simulink model "FirstAttempt_ColdEarth"  (R2018b)
settings: Solver=VariableStepAuto  StartTime=0.0  StopTime=time  RelTol=1e-3
values from neighbouring files (symbols this model uses):
  A_side = 2 * A_front    (= 0.02)    [MultipleNodes.m]    (also in OneNode.m)
  eps_f = 1    [OneNode.m]
  eps_l = 0.81    [OneNode.m]
  Qa_e = 0    [OneNode.m]
  Qi = 0.2*Qdiss    (= 0.6)    [OneNode.m]
  Qir_e = Wir_e *A_front *eps_b*REF    (= 1.8144)    [OneNode.m]
  QS_e = 0    [OneNode.m]
  sigma = 5.67e-8    (= 5.67e-08)    [MultipleNodes.m]    (also in OneNode.m)
  Tds = 4    [MultipleNodes.m]    (also in OneNode.m)
  Tsc_c = T_sc(1,1)    [OneNode.m]
libraries: fl_lib x19, nesl_utility x8
settings Model: Creator=aloisia  LastModifiedBy=aloisia

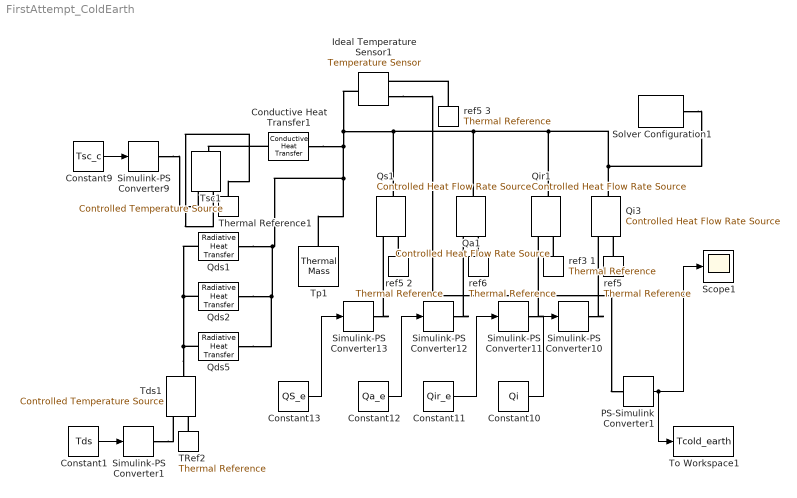
== system FirstAttempt_ColdEarth ==
  Conductive Heat Transfer1 : fl_lib/Thermal/Thermal Elements/Conductive Heat Transfer  area=0.005 m^2  thickness=0.01 m  th_cond=Gsc W/(m*K)  T_specify=off  T_priority=None  T=0 K  T_nominal_specify=off  T_nominal_unit=K  T_nominal_value=1  Q_specify=off  Q_priority=None  Q=0 J/s  Q_nominal_specify=off  Q_nominal_unit=W  Q_nominal_value=1
      settings: SourceProductName=Simscape
  Constant1 : Constant  Value=Tds
  Constant10 : Constant  Value=Qi
  Constant11 : Constant  Value=Qir_e
  Constant12 : Constant  Value=Qa_e
  Constant13 : Constant  Value=QS_e
  Constant9 : Constant  Value=Tsc_c
  Ideal Temperature Sensor1 : fl_lib/Thermal/Thermal Sensors/Temperature Sensor
  PS-Simulink Converter1 : nesl_utility/PS-Simulink Converter  PhysicalDomain=network_engine_domain  SubClassName=ps_output  LeftPortType=input  RightPortType=output  PseudoPeriodic=off  Frequencies=[]  Unit=1  AffineConversion=off
  Qa1 : fl_lib/Thermal/Thermal Sources/Controlled Heat Flow Rate Source
      settings: SourceProductName=Simscape
  Qds1 : fl_lib/Thermal/Thermal Elements/Radiative Heat Transfer  area=2*A_side m^2  rad_tr_coeff=sigma*eps_l W/(m^2*K^4)  T_specify=off  T_priority=None  T=0 K  T_nominal_specify=off  T_nominal_unit=K  T_nominal_value=1  Q_specify=off  Q_priority=None  Q=0 J/s  Q_nominal_specify=off  Q_nominal_unit=W  Q_nominal_value=1
      settings: SourceProductName=Simscape  SourceProductBaseCode=SS
  Qds2 : fl_lib/Thermal/Thermal Elements/Radiative Heat Transfer  area=A_front m^2  rad_tr_coeff=sigma*eps_f W/(m^2*K^4)  T_specify=off  T_priority=None  T=0 K  T_nominal_specify=off  T_nominal_unit=K  T_nominal_value=1  Q_specify=off  Q_priority=None  Q=0 J/s  Q_nominal_specify=off  Q_nominal_unit=W  Q_nominal_value=1
      settings: SourceProductName=Simscape  SourceProductBaseCode=SS
  Qds5 : fl_lib/Thermal/Thermal Elements/Radiative Heat Transfer  area=A_front m^2  rad_tr_coeff=sigma*eps_f W/(m^2*K^4)  T_specify=off  T_priority=None  T=0 K  T_nominal_specify=off  T_nominal_unit=K  T_nominal_value=1  Q_specify=off  Q_priority=None  Q=0 J/s  Q_nominal_specify=off  Q_nominal_unit=W  Q_nominal_value=1
      settings: SourceProductName=Simscape  SourceProductBaseCode=SS
  Qi3 : fl_lib/Thermal/Thermal Sources/Controlled Heat Flow Rate Source
      settings: SourceProductName=Simscape
  Qir1 : fl_lib/Thermal/Thermal Sources/Controlled Heat Flow Rate Source
      settings: SourceProductName=Simscape
  Qs1 : fl_lib/Thermal/Thermal Sources/Controlled Heat Flow Rate Source
      settings: SourceProductName=Simscape
  Scope1 : Scope
  Simulink-PS Converter{1,9..13} (6 alike) : nesl_utility/Simulink-PS Converter  PhysicalDomain=network_engine_domain  SubClassName=ps_input  LeftPortType=input  RightPortType=output  PseudoPeriodic=off  Frequencies=[]  NoiseDistribution=none  NoiseParameters=[]  Unit=1  AffineConversion=off  FilteringAndDerivatives=zero  SimscapeFilterOrder=1  InputFilterTimeConstant=0.001  UdotUserProvided=1
  Solver Configuration1 : nesl_utility/Solver Configuration  PhysicalDomain=network_engine_domain  SubClassName=solver  LeftPortType=input  RightPortType=generic  Tones=[]  Harmonics=[]  SimulateNoise=off  Profile=off  UseLocalSampling=off  EnableSwitchedLinearOptims=on  FrequencyDomain=off  UseCCode=off  RelTol=0.001  AbsTol=1e-06  MinStep=1e-09  ToWorkspace=off  RevertToSquareIcSolve=off  NumHomotopyIterations=100  PhasorMode=off  PhasorModeNumHarmonics=1  DoDC=off  ResidualTolerance=1e-09  UseLocalSolver=off  LocalSolverChoice=NE_BACKWARD_EULER_ADVANCER  LocalSolverSampleTime=0.001  DoFixedCost=off  MaxNonlinIter=3  MaxModeIter=2  LinearAlgebra=Full  EquationFormulation=NE_TIME_EF  DelaysMemoryBudget=1024  AutomaticFiltering=on  FilteringTimeConstant=0.001  PartitionStorageMethod=AS_NEEDED  PartitionMemoryBudget=1024
  TRef2 : fl_lib/Thermal/Thermal Elements/Thermal Reference
  Tds1 : fl_lib/Thermal/Thermal Sources/Controlled Temperature Source
      settings: SourceProductName=Simscape
  Thermal Reference1 : fl_lib/Thermal/Thermal Elements/Thermal Reference
  To Workspace1 : ToWorkspace  VariableName=Tcold_earth  SaveFormat=Timeseries  SampleTime=-1
  Tp1 : fl_lib/Thermal/Thermal Elements/Thermal Mass  mass=5 kg  sp_heat=447 J/kg/K  T_specify=on  T_priority=High  T=287.15 K  T_nominal_specify=off  T_nominal_unit=K  T_nominal_value=1  Q_specify=off  Q_priority=None  Q=0 J/s  Q_nominal_specify=off  Q_nominal_unit=W  Q_nominal_value=1
  Tsc1 : fl_lib/Thermal/Thermal Sources/Controlled Temperature Source
      settings: SourceProductName=Simscape
  ref3 1 : fl_lib/Thermal/Thermal Elements/Thermal Reference
  ref5 : fl_lib/Thermal/Thermal Elements/Thermal Reference
  ref5 2 : fl_lib/Thermal/Thermal Elements/Thermal Reference
  ref5 3 : fl_lib/Thermal/Thermal Elements/Thermal Reference
  ref6 : fl_lib/Thermal/Thermal Elements/Thermal Reference
  wires:
  Constant10/1 -> Simulink-PS Converter10/1
  Constant13/1 -> Simulink-PS Converter13/1
  Constant12/1 -> Simulink-PS Converter12/1
  Constant1/1 -> Simulink-PS Converter1/1
  Constant9/1 -> Simulink-PS Converter9/1
  Constant11/1 -> Simulink-PS Converter11/1
  PS-Simulink Converter1/1 -> To Workspace1/1, Scope1/1
  connections:
  Qds1/RConn1 -- Conductive Heat Transfer1/RConn1 -- Ideal Temperature Sensor1/LConn1 -- Solver Configuration1/RConn1 -- Qi3/LConn1 -- Qir1/LConn1 -- Qa1/LConn1 -- Qs1/LConn1 -- Tp1/LConn1 -- Qds5/RConn1 -- Qds2/RConn1
  Tds1/LConn1 -- Qds5/LConn1 -- Qds1/LConn1 -- Qds2/LConn1
  Simulink-PS Converter11/RConn1 -- Qir1/RConn1
  ref5 2/LConn1 -- Qs1/RConn2
  Simulink-PS Converter9/RConn1 -- Tsc1/RConn1
  Simulink-PS Converter13/RConn1 -- Qs1/RConn1
  Simulink-PS Converter10/RConn1 -- Qi3/RConn1
  ref5 3/LConn1 -- Ideal Temperature Sensor1/RConn1
  Conductive Heat Transfer1/LConn1 -- Tsc1/LConn1
  ref6/LConn1 -- Qa1/RConn2
  ref5/LConn1 -- Qi3/RConn2
  TRef2/LConn1 -- Tds1/RConn2
  Simulink-PS Converter1/RConn1 -- Tds1/RConn1
  Ideal Temperature Sensor1/RConn2 -- PS-Simulink Converter1/LConn1
  ref3 1/LConn1 -- Qir1/RConn2
  Thermal Reference1/LConn1 -- Tsc1/RConn2
  Simulink-PS Converter12/RConn1 -- Qa1/RConn1
